simulink model "UKFmini"  (R2024b)
settings: Solver=VariableStepAuto  StartTime=0.0  StopTime=10.0  RelTol=1e-3
libraries: simulink x1
settings Model: Creator=fanny  LastModifiedBy=fanny
settings DebuggingCC: UnderSpecifiedDimensionMsg=warning

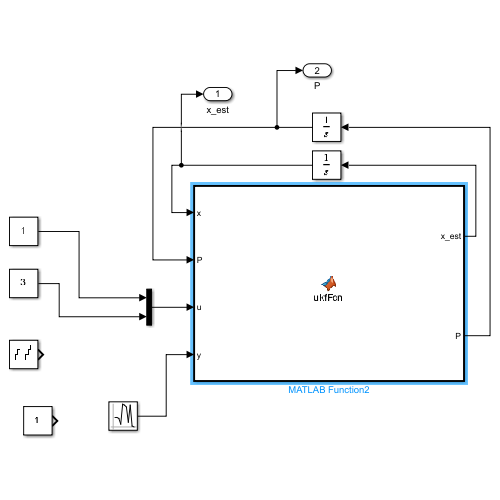
[thumbnail: Simulink's stored preview of the top-level diagram]
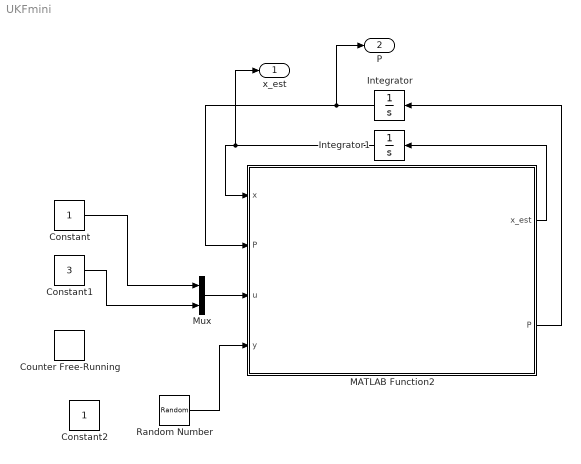
== system UKFmini ==
  Constant : Constant
  Constant1 : Constant  Value=3
  Constant2 : Constant
  Counter Free-Running : simulink/Sources/Counter Free-Running  NumBits=16  tsamp=-1
  Integrator : Integrator  InitialCondition=[0, 0;0, 0]
  Integrator1 : Integrator
  MATLAB Function2 : MATLAB Function  TreatAsAtomicUnit=on
  Mux : Mux  Inputs=2
  Random Number : RandomNumber  SampleTime=0.1
  x_est : Outport
  P : Outport  Port=2
  wires:
  MATLAB Function2/2(P) -> Integrator/1
  Integrator/1 -> P/1, MATLAB Function2/2("P ")
  MATLAB Function2/1(x_est) -> Integrator1/1
  Integrator1/1 -> x_est/1, MATLAB Function2/1(x)
  Constant/1 -> Mux/1
  Constant1/1 -> Mux/2
  Mux/1 -> MATLAB Function2/3(u)
  Random Number/1 -> MATLAB Function2/4(y)

== matlab function UKFmini/MATLAB Function2 ==
  data: x input; P input; u input; x_est output; y input; P output
function [x_est, P] = ukfFcn(x, P, u, y)
    % Unscented Kalman Filter Implementation
    % x: Current state estimate [position; velocity]
    % P: Current state covariance matrix
    % u: Control input (acceleration)
    % y: Measurement (position)
    % Q: Process noise covariance matrix
    % R: Measurement noise covariance matrix
    % x_est: Updated state estimate
    % P: Updated state covariance matrix
    x_est = zeros(2, 1);
    Q = [0.2 0.1;0.1 0.1];
    R = [0.1];
    u = [1;2];
    % Unscented Transform Parameters
    n = numel(x); % Number of states
    alpha = 1e-3; % Spread of sigma points
    kappa = 0;    % Secondary scaling parameter
    beta = 2;     % Optimal for Gaussian distributions
    lambda = alpha^2 * (n + kappa) - n; % Scaling parameter
    gamma = sqrt(n + lambda); % Scaling factor
    %L = chol(P, 'lower'); 

    % Generate Sigma Points
    % Sigma points are selected around the current mean x
    sigmaPoints = [x, ...
                   x + gamma * P(:, 1)', ...
                   x + gamma * P(:, 2)', ...
                   x - gamma * P(:, 1)', ...
                   x - gamma * P(:, 2)', ...
                   ];

    % Predict Step
    % Propagate each sigma point through the state transition function
    sigmaPointsPredicted = zeros(size(sigmaPoints));
    for i = 1:size(sigmaPoints, 2)
        sigmaPointsPredicted(:, i) = stateFcn(sigmaPoints(:, i), u);
    end

    % Predicted Mean and Covariance
    weightsMean = [0, 1 / 4, 1 / 4, 1 / 4, 1 / 4];
    weightsCov = weightsMean; 
    sigmaPointsPredicted = sigmaPointsPredicted(:,1:5);
    x_pred_1 = sigmaPointsPredicted(1,:) * weightsMean'; % Predicted state mean
    x_pred_2 = sigmaPointsPredicted(2,:) * weightsMean';
    x_pred = [x_pred_1; x_pred_2];
    P_pred = Q; % Initialize with process noise covariance
    for i = 1:size(sigmaPointsPredicted, 2)
        diff = sigmaPointsPredicted(:, i) - x_pred;
        P_pred = P_pred + weightsCov(i) * (diff * diff');
    end

    % Measurement Update Step
    % Transform the predicted sigma points through the measurement function
    sigmaPointsMeasurements = zeros(1, size(sigmaPointsPredicted, 2));
    for i = 1:size(sigmaPointsPredicted, 2)
        sigmaPointsMeasurements(:, i) = measurementFcn(sigmaPointsPredicted(:, i));
    end

    % Predicted Measurement Mean and Covariance
    y_pred = sigmaPointsMeasurements * weightsMean'; % Predicted measurement mean
    Pyy = R; % Initialize with measurement noise covariance
    for i = 1:size(sigmaPointsMeasurements, 2)
        diff = sigmaPointsMeasurements(:, i) - y_pred;
        Pyy = Pyy + weightsCov(i) * (diff * diff');
    end

    % Cross-Covariance between State and Measurement
    Pxy = zeros(n, 1);
    for i = 1:size(sigmaPointsPredicted, 2)
        stateDiff = sigmaPointsPredicted(:, i) - x_pred;
        measurementDiff = sigmaPointsMeasurements(:, i) - y_pred;
        Pxy = Pxy + weightsCov(i) * (stateDiff * measurementDiff');
    end

    % Kalman Gain
    K = Pxy / Pyy;

    % Update State and Covariance
    ys = y - y_pred;
    gain = K * ys;
    x_est = x_pred + gain; % Updated state estimate
    P = P_pred - K * Pyy * K'; % Updated covariance matrix
end


function x_next = stateFcn(x, u)
    % State transition function for the system.
    % x: Current state [position; velocity]
    % u: Control input (acceleration)
    % x_next: Next state
    
    dt = 0.1; % Time step
    A = [1 dt; 0 1]; % State transition matrix
    B = [0.5*dt^2; dt]; % Control input matrix
    
    % State evolution: x_next = A * x + B * u
    x_next = A * x + B .* u;
end


function y = measurementFcn(x)
    % Measurement function
    % x: Current state [position; velocity]
    % y: Measurement (position only in this example)
    
    % Assume we measure only position
    y = x(1);
end
